simulink model "modelo_final"  (R2013a)
settings: Solver=ode45  StartTime=0.0  StopTime=10.0  RelTol=1e-3
settings Model: Creator=jhona  LastModifiedBy=jhona

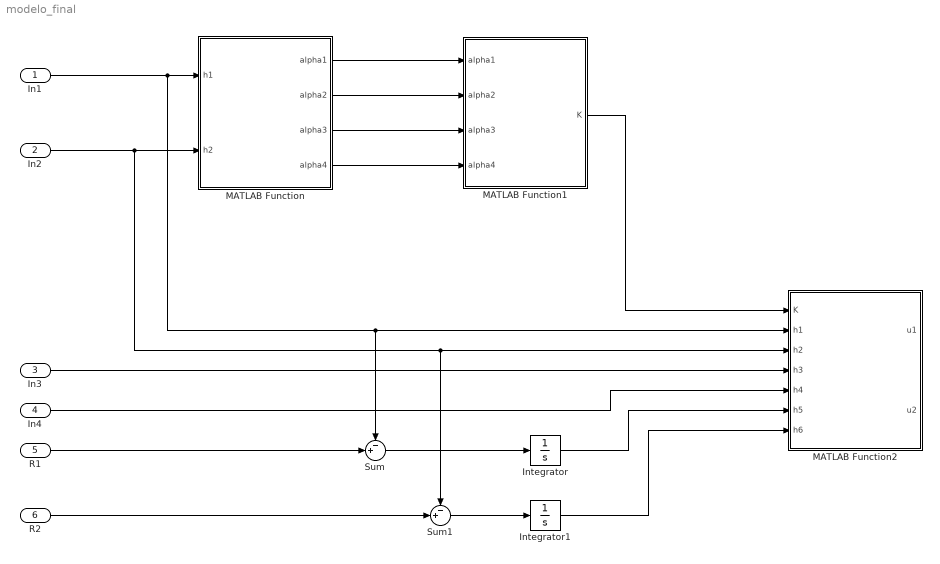
== system modelo_final ==
  In1 : Inport
  In2 : Inport  Port=2
  In3 : Inport  Port=3
  In4 : Inport  Port=4
  R1 : Inport  Port=5
  R2 : Inport  Port=6
  Integrator : Integrator
  Integrator1 : Integrator
  MATLAB Function : MATLAB Function  TreatAsAtomicUnit=on
  MATLAB Function1 : MATLAB Function  TreatAsAtomicUnit=on
  MATLAB Function2 : MATLAB Function  TreatAsAtomicUnit=on
  Sum : Sum  Inputs=-+|
  Sum1 : Sum  Inputs=-+|
  wires:
  In1/1 -> Sum/1, MATLAB Function2/2(h1), MATLAB Function/1(h1)
  In2/1 -> MATLAB Function2/3(h2), Sum1/1, MATLAB Function/2(h2)
  MATLAB Function/2(alpha2) -> MATLAB Function1/2(alpha2)
  MATLAB Function/1(alpha1) -> MATLAB Function1/1(alpha1)
  MATLAB Function/3(alpha3) -> MATLAB Function1/3(alpha3)
  MATLAB Function/4(alpha4) -> MATLAB Function1/4(alpha4)
  MATLAB Function1/1(K) -> MATLAB Function2/1(K)
  In4/1 -> MATLAB Function2/5(h4)
  In3/1 -> MATLAB Function2/4(h3)
  R2/1 -> Sum1/2
  R1/1 -> Sum/2
  Sum/1 -> Integrator/1
  Sum1/1 -> Integrator1/1
  Integrator/1 -> MATLAB Function2/6(h5)
  Integrator1/1 -> MATLAB Function2/7(h6)

== matlab function modelo_final/MATLAB Function1 ==
  data: alpha1 input; alpha2 input; alpha3 input; alpha4 input; K output
function K  = fcn(alpha1, alpha2, alpha3, alpha4)
%#codegen
k1 = 5;
k2 = 5;
k3 = 5;
k4 = 5;

K = alpha1*k1 + alpha2*k2 + alpha3*k3 + alpha4*k4;

== matlab function modelo_final/MATLAB Function ==
  data: h1 input; alpha1 output; h2 input; alpha2 output; alpha3 output; alpha4 output
function [alpha1, alpha2, alpha3, alpha4]  = fcn(h1,h2)
%#codegen

alpha1 = 0.25;
alpha2 = 0.25;
alpha3 = 0.25;
alpha4 = 0.25;

== matlab function modelo_final/MATLAB Function2 ==
  data: K input; h1 input; h2 input; h3 input; h4 input; h5 input; h6 input; u1 output; u2 output
function [u1, u2]  = fcn(K, h1, h2, h3, h4, h5, h6)
%#codegen
aux = K*[h1; h2; h3; h4; h5; h6];

u1 = aux(1);
u2 = aux(2);
